simulink model "mvariantsubsys"  (Simulink 7.6)
settings: Solver=FixedStepDiscrete  StartTime=0.0  StopTime=10.0  FixedStep=1  RelTol=1e-3
settings Model: Creator=mtocci  LastModifiedBy=mtocci
settings DataIOCC: LimitDataPoints=off  SaveFormat=StructureWithTime
settings OptimizationCC: InlineParams=on
settings DebuggingCC: StrictBusMsg=ErrorOnBusTreatedAsVector

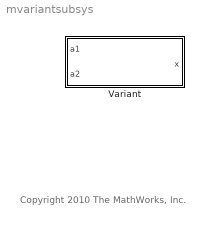
== system mvariantsubsys ==
  note: Copyright 2010 The MathWorks, Inc.
  Variant : Subsystem  Variant=on

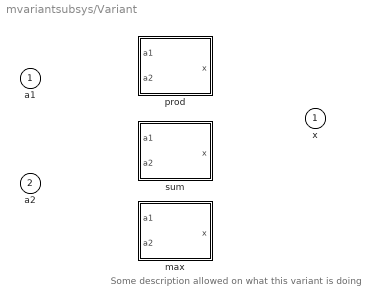
== system mvariantsubsys/Variant ==
  note: Some description allowed on what this variant is doing
  a1 : Inport
  a2 : Inport  Port=2
  max : Subsystem  VariantObject=varMax
  prod : Subsystem  VariantObject=varProd
  sum : Subsystem  VariantObject=varSum
  x : Outport  InitialOutput=0

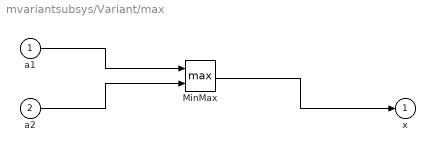
== system mvariantsubsys/Variant/max ==
  a1 : Inport
  a2 : Inport  Port=2
  MinMax : MinMax  Function=max  Inputs=2
  x : Outport  InitialOutput=0
  wires:
  a1/1 -> MinMax/1
  a2/1 -> MinMax/2
  MinMax/1 -> x/1

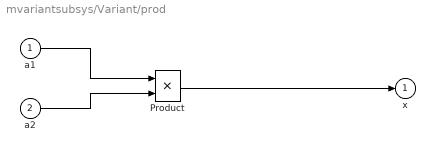
== system mvariantsubsys/Variant/prod ==
  a1 : Inport
  a2 : Inport  Port=2
  Product : Product  SaturateOnIntegerOverflow=on  RndMeth=Zero  InputSameDT=on  OutDataTypeStr=Inherit: Same as first input
  x : Outport  InitialOutput=0
  wires:
  Product/1 -> x/1
  a1/1 -> Product/1
  a2/1 -> Product/2

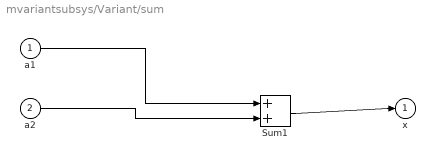
== system mvariantsubsys/Variant/sum ==
  a1 : Inport
  a2 : Inport  Port=2
  Sum1 : Sum  SaturateOnIntegerOverflow=on  InputSameDT=on  OutDataTypeStr=Inherit: Same as first input
  x : Outport  InitialOutput=0
  wires:
  Sum1/1 -> x/1
  a1/1 -> Sum1/1
  a2/1 -> Sum1/2
